simulink model "Example4_3_Model"  (R2018a)
settings: Solver=VariableStepAuto  StartTime=0.0  StopTime=10.0  RelTol=1e-3
libraries: simulink x1
settings Model: Creator=ewolbrec  LastModifiedBy=nalha
settings CodeAppCC: StateflowObjectComments=on

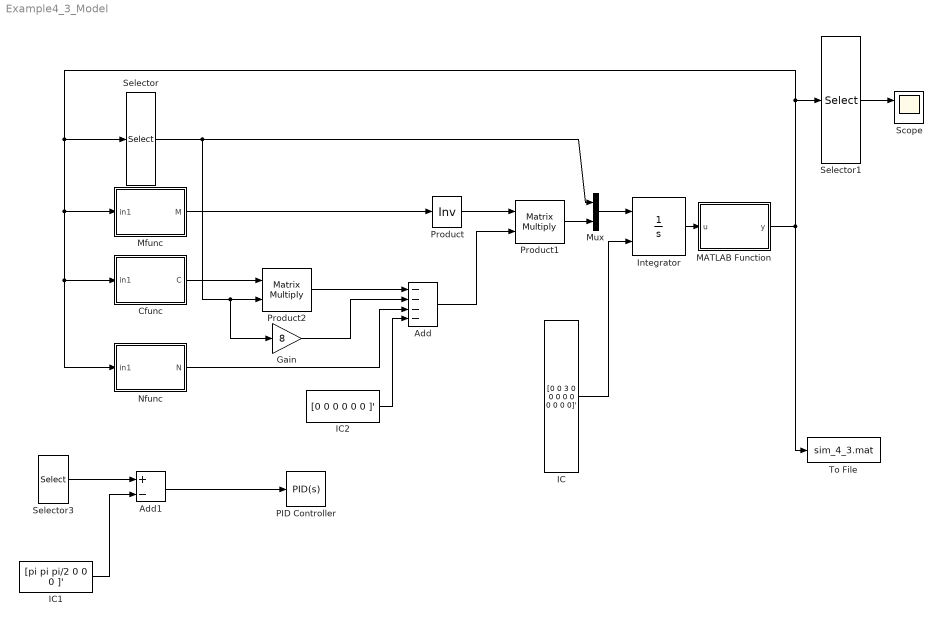
== system Example4_3_Model ==
  Add : Sum  Inputs=----
  Add1 : Sum  Inputs=+-
  Cfunc : MATLAB Function  TreatAsAtomicUnit=on
  Gain : Gain  Gain=8
  IC : Constant  Value=[0 0 3 0 0 0 0 0 0 0 0 0]'  VectorParams1D=off
  IC1 : Constant  Value=[pi pi pi/2 0 0 0 ]'  VectorParams1D=off
  IC2 : Constant  Value=[0 0 0 0 0 0 ]'  VectorParams1D=off
  Integrator : Integrator  InitialConditionSource=external
  MATLAB Function : MATLAB Function  TreatAsAtomicUnit=on
  Mfunc : MATLAB Function  TreatAsAtomicUnit=on
  Mux : Mux  Inputs=2
  Nfunc : MATLAB Function  TreatAsAtomicUnit=on
  PID Controller : simulink/Continuous/PID Controller  Controller=PID  TimeDomain=Continuous-time  SampleTime=-1  IntegratorMethod=Forward Euler  FilterMethod=Forward Euler  Form=Parallel  UseFilter=on  ControllerParametersSource=internal  P=100  I=10  D=30  N=100  InitialConditionSource=internal  InitialConditionForIntegrator=0  InitialConditionForFilter=0  ExternalReset=none  LimitOutput=off  UpperSaturationLimit=inf  LowerSaturationLimit=-inf  LinearizeAsGain=on  AntiWindupMode=none  Kb=1  TrackingMode=off  Kt=1  PParamMin=[]  PParamMax=[]  IParamMin=[]  IParamMax=[]  DParamMin=[]  DParamMax=[]  NParamMin=[]  NParamMax=[]  KbParamMin=[]  KbParamMax=[]  KtParamMin=[]  KtParamMax=[]  POutMin=[]  POutMax=[]  IOutMin=[]  IOutMax=[]  DOutMin=[]  DOutMax=[]  NOutMin=[]  NOutMax=[]  KbOutMin=[]  KbOutMax=[]  KtOutMin=[]  KtOutMax=[]  IntegratorOutMin=[]  IntegratorOutMax=[]  FilterOutMin=[]  FilterOutMax=[]  SumOutMin=[]  SumOutMax=[]  SumI1OutMin=[]  SumI1OutMax=[]  SumI2OutMin=[]  SumI2OutMax=[]  SumI3OutMin=[]  SumI3OutMax=[]  SumDOutMin=[]  SumDOutMax=[]  SaturationOutMin=[]  SaturationOutMax=[]  IntegratorContinuousStateAttributes=''  IntegratorStateMustResolveToSignalObject=off  IntegratorRTWStateStorageClass=Auto  FilterContinuousStateAttributes=''  FilterStateMustResolveToSignalObject=off  FilterRTWStateStorageClass=Auto  DifferentiatorICPrevScaledInput=0  DifferentiatorOutMin=[]  DifferentiatorOutMax=[]  FilterDiffOutCoefMin=[]  FilterDiffOutCoefMax=[]  SumDenOutMin=[]  SumDenOutMax=[]  SumNumOutMin=[]  SumNumOutMax=[]  ReciprocalOutMin=[]  ReciprocalOutMax=[]  DivideOutMin=[]  DivideOutMax=[]  TunerSelectOption=Transfer Function Based (PID Tuner App)
  Product : Product  Inputs=/  Multiplication=Matrix(*)
  Product1 : Product  Inputs=**  Multiplication=Matrix(*)
  Product2 : Product  Inputs=**  Multiplication=Matrix(*)
  Scope : Scope  NumInputPorts=2
  Selector : Selector  InputPortWidth=12  IndexOptions=Index vector (dialog)  Indices=[7 8 9 10 11 12]  OutputSizes=1
  Selector1 : Selector  InputPortWidth=12  IndexOptions=Index vector (dialog)  Indices=[1 2 3 4 5 6]  OutputSizes=1
  Selector3 : Selector  InputPortWidth=12  IndexOptions=Index vector (dialog)  Indices=[1 2 3 4 5 6]  OutputSizes=1
  To File : ToFile  Filename=sim_4_3.mat  SampleTime=1/30
  wires:
  Mfunc/1(M) -> Product/1
  Mux/1 -> Integrator/1
  Product1/1 -> Mux/2
  Selector/1 -> Gain/1, Product2/2, Mux/1
  Cfunc/1(C) -> Product2/1
  Product/1 -> Product1/1
  Gain/1 -> Add/2
  Product2/1 -> Add/1
  Nfunc/1(N) -> Add/3
  Add/1 -> Product1/2
  IC/1 -> Integrator/2
  Selector1/1 -> Scope/1
  Selector3/1 -> Add1/1
  IC1/1 -> Add1/2
  Add1/1 -> PID Controller/1
  IC2/1 -> Add/4
  Integrator/1 -> MATLAB Function/1(u)
  MATLAB Function/1(y) -> To File/1, Mfunc/1(in1), Cfunc/1(in1), Nfunc/1(in1), Selector/1, Selector1/1

== matlab function Example4_3_Model/Cfunc ==
  data: in1 input; C output
function C = Cfunc(in1)
%#codegen

%    This function was generated by the Symbolic Math Toolbox version 8.1.
%    08-May-2018 14:20:51

th4 = in1(4,:);
th5 = in1(5,:);
th6 = in1(6,:);
th4d = in1(10,:);
th5d = in1(11,:);
th6d = in1(12,:);
t2 = cos(th4);
t3 = cos(th5);
t4 = sin(th4);
t5 = cos(th6);
t6 = sin(th5);
t7 = sin(th6);
t8 = t2.*t3.*t7.*th4d.*(2.7e1./8.0);
t9 = t2.*t5.*t6.*th4d.*(2.7e1./8.0);
t10 = t3.*t4.*t5.*th5d.*(2.7e1./8.0);
t11 = t3.*t4.*t5.*th6d.*(2.7e1./8.0);
t12 = t3.*t4.*t7.*th4d.*(2.7e1./8.0);
t13 = t4.*t5.*t6.*th4d.*(2.7e1./8.0);
t14 = t2.*t6.*t7.*th5d.*(2.7e1./8.0);
t15 = t2.*t6.*t7.*th6d.*(2.7e1./8.0);
t16 = th5+th6;
t17 = sin(t16);
t18 = th5.*2.0;
t19 = th6.*2.0;
t20 = t18+t19;
t21 = sin(t20);
t22 = t18+th6;
t23 = sin(t22);
t24 = sin(t18);
t25 = cos(t16);
t26 = th5d+th6d;
t27 = t21.*3.3e1;
C = reshape([0.0,0.0,0.0,0.0,0.0,0.0,0.0,0.0,0.0,0.0,0.0,0.0,0.0,0.0,0.0,0.0,0.0,0.0,t2.*th4d.*(-2.7e1./1.0e1)+t3.*t4.*th4d.*(8.1e1./8.0)+t2.*t6.*th5d.*(8.1e1./8.0)+t3.*t4.*t5.*th4d.*(2.7e1./8.0)+t2.*t3.*t7.*th5d.*(2.7e1./8.0)+t2.*t3.*t7.*th6d.*(2.7e1./8.0)+t2.*t5.*t6.*th5d.*(2.7e1./8.0)+t2.*t5.*t6.*th6d.*(2.7e1./8.0)-t4.*t6.*t7.*th4d.*(2.7e1./8.0),t4.*th4d.*(-2.7e1./1.0e1)-t2.*t3.*th4d.*(8.1e1./8.0)+t4.*t6.*th5d.*(8.1e1./8.0)-t2.*t3.*t5.*th4d.*(2.7e1./8.0)+t2.*t6.*t7.*th4d.*(2.7e1./8.0)+t3.*t4.*t7.*th5d.*(2.7e1./8.0)+t3.*t4.*t7.*th6d.*(2.7e1./8.0)+t4.*t5.*t6.*th5d.*(2.7e1./8.0)+t4.*t5.*t6.*th6d.*(2.7e1./8.0),0.0,t7.*th6d.*(-2.7e1./3.2e1)-t21.*th5d.*5.56875e-1-t21.*th6d.*5.56875e-1-t23.*th5d.*(2.7e1./1.6e1)-t23.*th6d.*(2.7e1./3.2e1)-t24.*th5d.*2.244375,th4d.*(t23.*1.0e2+t24.*1.33e2+t27).*1.6875e-2,th4d.*(t7.*5.0e1+t23.*5.0e1+t27).*1.6875e-2,t8+t9+t10+t11+t2.*t6.*th4d.*(8.1e1./8.0)+t3.*t4.*th5d.*(8.1e1./8.0)-t4.*t6.*t7.*th5d.*(2.7e1./8.0)-t4.*t6.*t7.*th6d.*(2.7e1./8.0),t12+t13+t14+t15-t2.*t3.*th5d.*(8.1e1./8.0)+t4.*t6.*th4d.*(8.1e1./8.0)-t2.*t3.*t5.*th5d.*(2.7e1./8.0)-t2.*t3.*t5.*th6d.*(2.7e1./8.0),t6.*th5d.*(8.1e1./8.0)+t17.*th5d.*(2.7e1./8.0)+t17.*th6d.*(2.7e1./8.0),t3.*th5d.*(-8.1e1./8.0e1)-t21.*th4d.*5.56875e-1-t23.*th4d.*(2.7e1./1.6e1)-t24.*th4d.*2.244375-t25.*th5d.*(2.7e1./8.0e1)-t25.*th6d.*(2.7e1./8.0e1),t7.*th6d.*(-2.7e1./1.6e1),t7.*th5d.*(2.7e1./1.6e1),t8+t9+t10+t11-t4.*t6.*t7.*th5d.*(2.7e1./8.0)-t4.*t6.*t7.*th6d.*(2.7e1./8.0),t12+t13+t14+t15-t2.*t3.*t5.*th5d.*(2.7e1./8.0)-t2.*t3.*t5.*th6d.*(2.7e1./8.0),t17.*t26.*(2.7e1./8.0),t7.*th4d.*(-2.7e1./3.2e1)-t21.*th4d.*5.56875e-1-t23.*th4d.*(2.7e1./3.2e1)-t25.*th5d.*(2.7e1./8.0e1)-t25.*th6d.*(2.7e1./8.0e1),t7.*t26.*(-2.7e1./1.6e1),0.0],[6,6]);

== matlab function Example4_3_Model/Mfunc ==
  data: in1 input; M output
function M = Mfunc(in1)
%#codegen

%    This function was generated by the Symbolic Math Toolbox version 8.1.
%    08-May-2018 14:20:51

th4 = in1(4,:);
th5 = in1(5,:);
th6 = in1(6,:);
t2 = cos(th4);
t3 = cos(th5);
t4 = sin(th4);
t5 = sin(th5);
t6 = th5+th6;
t7 = sin(t6);
t8 = sin(th6);
t9 = cos(th6);
t10 = t5.*3.0;
t11 = t7+t10;
t12 = cos(t6);
t13 = t2.*t5.*t8.*(2.7e1./8.0);
t14 = t4.*(-2.7e1./1.0e1)+t13-t2.*t3.*(8.1e1./8.0)-t2.*t3.*t9.*(2.7e1./8.0);
t15 = t2.*(2.7e1./1.0e1);
t16 = t4.*t5.*t8.*(2.7e1./8.0);
t17 = t15+t16-t3.*t4.*(8.1e1./8.0)-t3.*t4.*t9.*(2.7e1./8.0);
t18 = th5.*2.0;
t19 = t4.*t11.*(2.7e1./8.0);
t24 = t12.*(2.7e1./8.0);
t20 = t3.*(-8.1e1./8.0)-t24;
t25 = t7.*(2.7e1./8.0e1);
t21 = t5.*(-8.1e1./8.0e1)-t25;
t22 = t9.*(2.7e1./1.6e1);
t23 = t4.*t7.*(2.7e1./8.0);
t26 = t22+9.07e2./8.0e2;
M = reshape([7.83e2./5.0,0.0,0.0,t14,t19,t23,0.0,7.83e2./5.0,0.0,t17,t2.*t11.*(-2.7e1./8.0),t2.*t7.*(-2.7e1./8.0),0.0,0.0,7.83e2./5.0,0.0,t20,-t24,t14,t17,0.0,t22+cos(t18+th6.*2.0).*5.56875e-1+cos(t18+th6).*(2.7e1./1.6e1)+cos(t18).*2.244375+6.57125,t21,-t25,t19,t2.*t11.*(-2.7e1./8.0),t20,t21,t9.*(2.7e1./8.0)+5.6425,t26,t23,t2.*t7.*(-2.7e1./8.0),t12.*(-2.7e1./8.0),t7.*(-2.7e1./8.0e1),t26,9.07e2./8.0e2],[6,6]);

== matlab function Example4_3_Model/Nfunc ==
  data: in1 input; N output
function N = Nfunc(in1)
%#codegen

%    This function was generated by the Symbolic Math Toolbox version 8.1.
%    08-May-2018 14:20:51

th5 = in1(5,:);
th6 = in1(6,:);
t2 = th5+th6;
t3 = cos(t2);
N = [0.0;0.0;1.566e3;0.0;t3.*(-1.35e2./4.0)-cos(th5).*(4.05e2./4.0);t3.*(-1.35e2./4.0)];

== matlab function Example4_3_Model/MATLAB Function ==
  data: u input; y output
function y = floorSim(u)
% Simulate floor in z-dir so we don't lose our robot

    y = u; %pass through vector

    
    % edit only if we're going through the floor
    if u(3) < 0 && u(9) < 0
        y(9) = -.7*u(9); %Flip sign and reduce velocity by arbitrary amount
    end
end
